simulink model "Simu_Grua"  (R2022a)
settings: Solver=VariableStepAuto  StartTime=0.0  StopTime=50  RelTol=1e-3
values from neighbouring files (symbols this model uses):
  K = Ks(1:4)    [Copy_of_grua.m]    (also in workspace_variables - copia.mat = [9.76340486456 -5.82004184641 1.0541659868 0.253205039146])
libraries: cstblocks x5, simulink x1
settings Model: Creator=carlo  LastModifiedBy=carlo

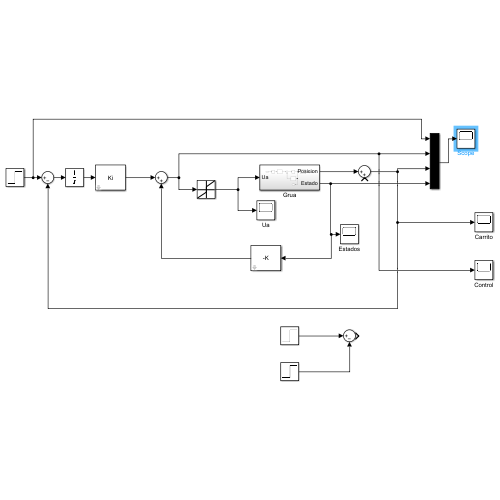
[thumbnail: Simulink's stored preview of the top-level diagram]
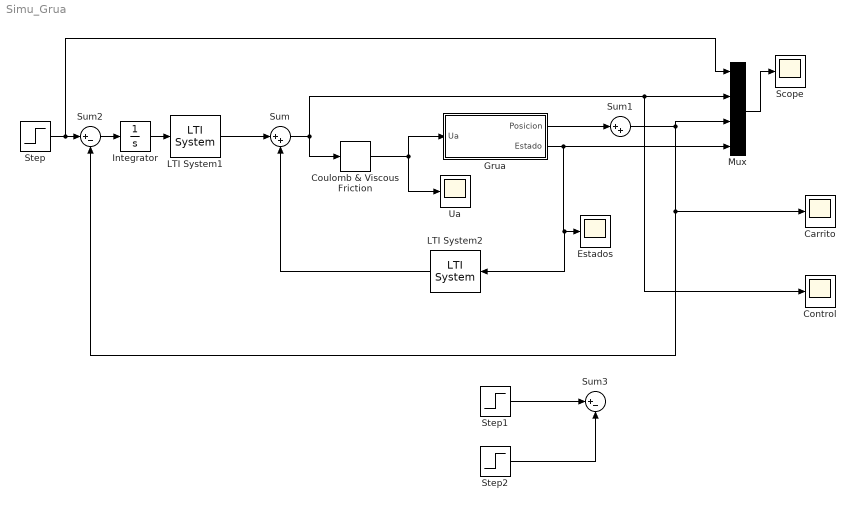
== system Simu_Grua ==
  Carrito : Scope
  Control : Scope
  Coulomb & Viscous Friction : simulink/Discontinuities/Coulomb & Viscous Friction  offset=[0.4]  gain=1
  Estados : Scope
  Grua : Subsystem
  Integrator : Integrator
  LTI System1 : cstblocks/LTI System  sys=Ki  IC=[]
  LTI System2 : cstblocks/LTI System  sys=-K  IC=[]
  Mux : Mux
  Scope : Scope
  Step : Step  After=0.5  SampleTime=0
  Step1 : Step  Time=0.1  After=8  SampleTime=0
  Step2 : Step  Time=0.1  After=10  SampleTime=0
  Sum : Sum  Inputs=|++
  Sum1 : Sum  Inputs=|++
  Sum2 : Sum  Inputs=|+-
  Sum3 : Sum  Inputs=|+-
  Ua : Scope
  wires:
  Coulomb & Viscous Friction/1 -> Grua/1(Ua), Ua/1
  Sum/1 -> Mux/2, Control/1, Coulomb & Viscous Friction/1
  Grua/2(Estado) -> LTI System2/1, Estados/1, Mux/4
  Grua/1(Posicion) -> Sum1/1
  Sum1/1 -> Carrito/1, Sum2/2, Mux/3
  Step/1 -> Sum2/1, Mux/1
  LTI System2/1 -> Sum/2
  Integrator/1 -> LTI System1/1
  Sum2/1 -> Integrator/1
  Step1/1 -> Sum3/1
  Step2/1 -> Sum3/2
  LTI System1/1 -> Sum/1
  Mux/1 -> Scope/1

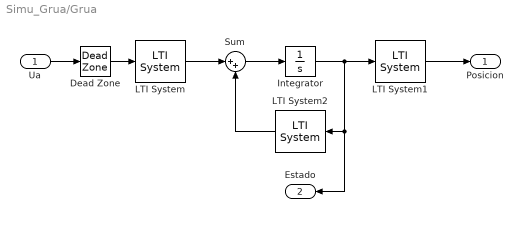
== system Simu_Grua/Grua ==
  Ua : Inport
  Dead Zone : DeadZone  UpperValue=0.6
  Integrator : Integrator
  LTI System : cstblocks/LTI System  sys=B  IC=[]
  LTI System1 : cstblocks/LTI System  sys=C  IC=[]
  LTI System2 : cstblocks/LTI System  sys=A  IC=[]
  Sum : Sum  Inputs=|++
  Posicion : Outport
  Estado : Outport  Port=2
  wires:
  LTI System/1 -> Sum/1
  Sum/1 -> Integrator/1
  Integrator/1 -> Estado/1, LTI System2/1, LTI System1/1
  LTI System1/1 -> Posicion/1
  LTI System2/1 -> Sum/2
  Dead Zone/1 -> LTI System/1
  Ua/1 -> Dead Zone/1
